simulink model "power_PVArray_PartialShading9x9new"  (R2019a)
settings: Solver=VariableStepAuto  StartTime=0.0  StopTime=9  FixedStep=Ts_Power  RelTol=1e-4
PreLoadFcn:
  | Ts_Power=50e-6;
  | Slope_Vdc=1;
InitFcn:
  | Ts_Power=50e-6;
  | Tc=1e-5;%break algebraic loop time constant
  | BlockName=[gcs,'/PV module 1'];
  | ModuleName=get_param(BlockName,'ModuleName');
  | Voc1=str2num(get_param(BlockName,'Voc'));
  | Nser1=str2num(get_param(BlockName,'Nser'));
  | Slope_Vdc=Nser1*Voc1;
StopFcn:
  | if exist('I','var') && exist('V','var')
  |    figure(1)
  |    clf
  |    n=find(I>=0);
  |    n=n(end);
  |    Vglobal=V(1:n);
  |    Iglobal=I(1:n);
  | 
  | 
  |    Pglobal=Vglobal.*Iglobal;
  |    n=find(Pglobal==max(Pglobal));
  |    Pmax=Pglobal(n);
  |    Vmp=Vglobal(n);
  |    Imp=Iglobal(n);
  | 
  | 
  |    subplot(211)
  |    plot(Vglobal, Iglobal,Vmp,Imp,'or')
  |    ylabel('Current (A)')
  |    title(sprintf('Global I-V & P-V characteristics\n %s' ,ModuleName))
  | 
  | 
  |    subplot(212)
  |    plot(Vglobal, Pglobal,Vmp,Pmax,'or')
  |    ylabel('Power (W)')
  |    xlabel('Voltage (V)')
  | end
undefined symbols (not defined in the file or in its folder): Irr
libraries: powerlib x85, re_lib x81, simulink x1
Description:
  | Copyright 2008-2019 The MathWorks, Inc.
settings Model: Creator=MathWorks  LastModifiedBy=makis
settings SolverCC: AlgebraicLoopSolver=LineSearch
settings DataIOCC: LimitDataPoints=on  SaveFormat=Array  SignalLoggingSaveFormat=ModelDataLogs  ReturnWorkspaceOutputs=off
settings OptimizationCC: ExpressionDepthLimit=2147483647  LifeSpan=inf
settings DebuggingCC: UnderspecifiedInitializationDetection=Classic  MergeDetectMultiDrivingBlocksExec=none  SolverPrmCheckMsg=warning  FcnCallInpInsideContextMsg=warning  AllowSymbolicDim=off  StateNameClashWarn=warning  SFUnexpectedBacktrackingDiag=warning  SFNoUnconditionalDefaultTransitionDiag=warning  SFExecutionAtInitializationDiag=none  ArithmeticOperatorsInVariantConditions=warning
settings HardwareCC: ProdBitPerPointer=32  ProdBitPerSizeT=32  ProdBitPerPtrDiffT=32  ProdLargestAtomicFloat=None  ProdIntDivRoundTo=Undefined  ProdEndianess=Unspecified  ProdWordSize=32  ProdHWDeviceType=32-bit Generic
settings ModelReferenceCC: PropagateSignalLabelsOutOfModel=off
settings SFSimCC: SimUseLocalCustomCode=off
settings RTWCC: RTWUseLocalCustomCode=off
settings CodeAppCC: StateflowObjectComments=on
settings GRTTargetCC: TargetLangStandard=C89/C90 (ANSI)  GeneratePreprocessorConditionals=Disable all  CombineOutputUpdateFcns=off  GRTInterface=on
settings ConfigComp: CovMetricSettings=dw  CovHtmlReporting=on  CovSaveCumulativeToWorkspaceVar=on  CovSaveSingleToWorkspaceVar=on  CovExternalEMLEnable=off  CovSFcnEnable=off
settings SimscapeCC: SimscapeNormalizeSystem=off

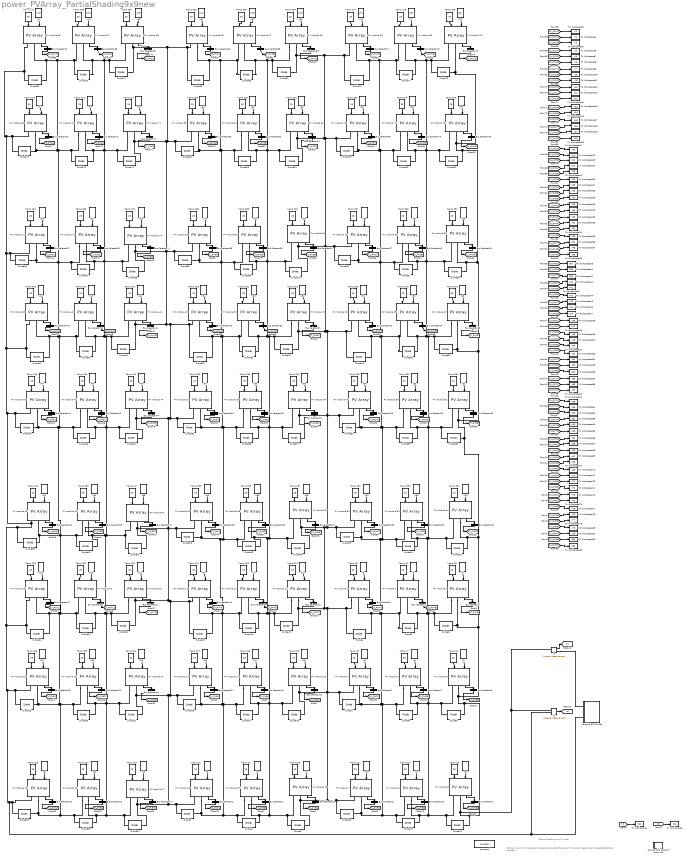
== system power_PVArray_PartialShading9x9new ==
  note: Global I-V and P-V characteristic are displayed at the end of simulation
      | (see Model Properties/Callback StopFcn)
  note: Partial Shading of a PV Array
  Bus Selector{1..81} (81 alike) : BusSelector  OutputSignals=V_PV,I_PV  OutputAsBus=on
  Diode{1..81} (81 alike) : powerlib/Power Electronics/Diode  Ron=0.001  Lon=0  Vf=0.7  IC=0  UseSnubber=off  Rs=1e5*inf  Cs=inf  Measurements=off
      settings: SourceProductName=Simscape Electrical
  Double click here for more info : Subsystem
      settings: OpenFcn=showdemo(bdroot(gcb))
      mask Display: disp('?')
  I1 : powerlib/Measurements/Current Measurement  PhasorSimulation=off  OutputType=Complex  PSBequivalent=0
      settings: SourceProductName=Simscape Electrical
  Ir1 : Constant  Value=Irr(78)
  Ir10 : Constant  Value=Irr(81)
  Ir11 : Constant  Value=Irr(80)
  Ir12 : Constant  Value=Irr(79)
  Ir13 : Constant  Value=Irr(60)
  Ir14 : Constant  Value=Irr(59)
  Ir15 : Constant  Value=Irr(58)
  Ir16 : Constant  Value=Irr(69)
  Ir17 : Constant  Value=Irr(68)
  Ir18 : Constant  Value=Irr(67)
  Ir19 : Constant  Value=Irr(75)
  Ir2 : Constant  Value=Irr(77)
  Ir20 : Constant  Value=Irr(74)
  Ir21 : Constant  Value=Irr(73)
  Ir22 : Constant  Value=Irr(57)
  Ir23 : Constant  Value=Irr(56)
  Ir24 : Constant  Value=Irr(55)
  Ir25 : Constant  Value=Irr(66)
  Ir26 : Constant  Value=Irr(65)
  Ir27 : Constant  Value=Irr(64)
  Ir28 : Constant  Value=Irr(51)
  Ir29 : Constant  Value=Irr(54)
  Ir3 : Constant  Value=Irr(76)
  Ir30 : Constant  Value=Irr(53)
  Ir31 : Constant  Value=Irr(52)
  Ir32 : Constant  Value=Irr(33)
  Ir33 : Constant  Value=Irr(32)
  Ir34 : Constant  Value=Irr(31)
  Ir35 : Constant  Value=Irr(42)
  Ir36 : Constant  Value=Irr(41)
  Ir37 : Constant  Value=Irr(40)
  Ir38 : Constant  Value=Irr(48)
  Ir39 : Constant  Value=Irr(50)
  Ir4 : Constant  Value=Irr(63)
  Ir40 : Constant  Value=Irr(47)
  Ir41 : Constant  Value=Irr(46)
  Ir42 : Constant  Value=Irr(30)
  Ir43 : Constant  Value=Irr(29)
  Ir44 : Constant  Value=Irr(28)
  Ir45 : Constant  Value=Irr(39)
  Ir46 : Constant  Value=Irr(38)
  Ir47 : Constant  Value=Irr(37)
  Ir48 : Constant  Value=Irr(49)
  Ir49 : Constant  Value=Irr(36)
  Ir5 : Constant  Value=Irr(62)
  Ir50 : Constant  Value=Irr(35)
  Ir51 : Constant  Value=Irr(34)
  Ir52 : Constant  Value=Irr(45)
  Ir53 : Constant  Value=Irr(44)
  Ir54 : Constant  Value=Irr(43)
  Ir55 : Constant  Value=Irr(24)
  Ir56 : Constant  Value=Irr(27)
  Ir57 : Constant  Value=Irr(26)
  Ir58 : Constant  Value=Irr(25)
  Ir59 : Constant  Value=Irr(6)
  Ir6 : Constant  Value=Irr(61)
  Ir60 : Constant  Value=Irr(5)
  Ir61 : Constant  Value=Irr(4)
  Ir62 : Constant  Value=Irr(15)
  Ir63 : Constant  Value=Irr(14)
  Ir64 : Constant  Value=Irr(13)
  Ir65 : Constant  Value=Irr(21)
  Ir66 : Constant  Value=Irr(23)
  Ir67 : Constant  Value=Irr(20)
  Ir68 : Constant  Value=Irr(19)
  Ir69 : Constant  Value=Irr(3)
  Ir7 : Constant  Value=Irr(72)
  Ir70 : Constant  Value=Irr(2)
  Ir71 : Constant  Value=Irr(1)
  Ir72 : Constant  Value=Irr(12)
  Ir73 : Constant  Value=Irr(11)
  Ir74 : Constant  Value=Irr(10)
  Ir75 : Constant  Value=Irr(22)
  Ir76 : Constant  Value=Irr(9)
  Ir77 : Constant  Value=Irr(8)
  Ir78 : Constant  Value=Irr(7)
  Ir79 : Constant  Value=Irr(18)
  Ir8 : Constant  Value=Irr(71)
  Ir80 : Constant  Value=Irr(17)
  Ir81 : Constant  Value=Irr(16)
  Ir9 : Constant  Value=Irr(70)
  PV module {1..81} (81 alike) : re_lib/Solar/PV Array  Npar=1  Nser=1  PlotType=array @ 25 deg.C & specified irradiances  S_vec="[ 1000  500  100 ]"  Temp_C_vec="[ 45 25  ]"  ModuleName=Mitsubishi Electric PV-MLU255HC  PlotWhenSelected=off  Pm=255.216  Ncell=60  Voc=37.8  Isc=8.89  Vm=31.2  Im=8.18  beta_Voc_pc=-0.38701  alpha_Isc_pc=0.104  beta_Voc=-0.14629  alpha_Isc=0.009246  IL=8.9065  I0=7.8419e-10  nI=1.0608  Rsh=114.9388  Rs=0.21303  BAL=on  Tc=Tc  Tfilter=5e-5
      settings: SourceProductName=Simscape Electrical
  Temp C{1..81} (81 alike) : Constant  Value=25
  To Workspace1 : ToWorkspace  VariableName=Vtot  SampleTime=1e-3
  To Workspace10 : ToWorkspace  VariableName=V8  SampleTime=1e-3
  To Workspace11 : ToWorkspace  VariableName=V9  SampleTime=1e-3
  To Workspace12 : ToWorkspace  VariableName=V10  SampleTime=1e-3
  To Workspace13 : ToWorkspace  VariableName=V11  SampleTime=1e-3
  To Workspace14 : ToWorkspace  VariableName=V12  SampleTime=1e-3
  To Workspace15 : ToWorkspace  VariableName=V13  SampleTime=1e-3
  To Workspace16 : ToWorkspace  VariableName=V14  SampleTime=1e-3
  To Workspace17 : ToWorkspace  VariableName=V15  SampleTime=1e-3
  To Workspace18 : ToWorkspace  VariableName=V16  SampleTime=1e-3
  To Workspace19 : ToWorkspace  VariableName=V17  SampleTime=1e-3
  To Workspace2 : ToWorkspace  VariableName=Itot  SampleTime=1e-3
  To Workspace20 : ToWorkspace  VariableName=V18  SampleTime=1e-3
  To Workspace21 : ToWorkspace  VariableName=V19  SampleTime=1e-3
  To Workspace22 : ToWorkspace  VariableName=V20  SampleTime=1e-3
  To Workspace23 : ToWorkspace  VariableName=V21  SampleTime=1e-3
  To Workspace24 : ToWorkspace  VariableName=V22  SampleTime=1e-3
  To Workspace25 : ToWorkspace  VariableName=V23  SampleTime=1e-3
  To Workspace26 : ToWorkspace  VariableName=V24  SampleTime=1e-3
  To Workspace27 : ToWorkspace  VariableName=V25  SampleTime=1e-3
  To Workspace28 : ToWorkspace  VariableName=V26  SampleTime=1e-3
  To Workspace29 : ToWorkspace  VariableName=V27  SampleTime=1e-3
  To Workspace3 : ToWorkspace  VariableName=V1  SampleTime=1e-3
  To Workspace30 : ToWorkspace  VariableName=V28  SampleTime=1e-3
  To Workspace31 : ToWorkspace  VariableName=V29  SampleTime=1e-3
  To Workspace32 : ToWorkspace  VariableName=V30  SampleTime=1e-3
  To Workspace33 : ToWorkspace  VariableName=V31  SampleTime=1e-3
  To Workspace34 : ToWorkspace  VariableName=V32  SampleTime=1e-3
  To Workspace35 : ToWorkspace  VariableName=V33  SampleTime=1e-3
  To Workspace36 : ToWorkspace  VariableName=V34  SampleTime=1e-3
  To Workspace37 : ToWorkspace  VariableName=V35  SampleTime=1e-3
  To Workspace38 : ToWorkspace  VariableName=V36  SampleTime=1e-3
  To Workspace39 : ToWorkspace  VariableName=V37  SampleTime=1e-3
  To Workspace4 : ToWorkspace  VariableName=V2  SampleTime=1e-3
  To Workspace40 : ToWorkspace  VariableName=V38  SampleTime=1e-3
  To Workspace41 : ToWorkspace  VariableName=V39  SampleTime=1e-3
  To Workspace42 : ToWorkspace  VariableName=V40  SampleTime=1e-3
  To Workspace43 : ToWorkspace  VariableName=V41  SampleTime=1e-3
  To Workspace44 : ToWorkspace  VariableName=V42  SampleTime=1e-3
  To Workspace45 : ToWorkspace  VariableName=V43  SampleTime=1e-3
  To Workspace46 : ToWorkspace  VariableName=V44  SampleTime=1e-3
  To Workspace47 : ToWorkspace  VariableName=V45  SampleTime=1e-3
  To Workspace48 : ToWorkspace  VariableName=V46  SampleTime=1e-3
  To Workspace49 : ToWorkspace  VariableName=V47  SampleTime=1e-3
  To Workspace5 : ToWorkspace  VariableName=V3  SampleTime=1e-3
  To Workspace50 : ToWorkspace  VariableName=V48  SampleTime=1e-3
  To Workspace51 : ToWorkspace  VariableName=V49  SampleTime=1e-3
  To Workspace52 : ToWorkspace  VariableName=V50  SampleTime=1e-3
  To Workspace53 : ToWorkspace  VariableName=V51  SampleTime=1e-3
  To Workspace54 : ToWorkspace  VariableName=V52  SampleTime=1e-3
  To Workspace55 : ToWorkspace  VariableName=V53  SampleTime=1e-3
  To Workspace56 : ToWorkspace  VariableName=V54  SampleTime=1e-3
  To Workspace57 : ToWorkspace  VariableName=V55  SampleTime=1e-3
  To Workspace58 : ToWorkspace  VariableName=V56  SampleTime=1e-3
  To Workspace59 : ToWorkspace  VariableName=V57  SampleTime=1e-3
  To Workspace6 : ToWorkspace  VariableName=V4  SampleTime=1e-3
  To Workspace60 : ToWorkspace  VariableName=V58  SampleTime=1e-3
  To Workspace61 : ToWorkspace  VariableName=V59  SampleTime=1e-3
  To Workspace62 : ToWorkspace  VariableName=V60  SampleTime=1e-3
  To Workspace63 : ToWorkspace  VariableName=V61  SampleTime=1e-3
  To Workspace64 : ToWorkspace  VariableName=V62  SampleTime=1e-3
  To Workspace65 : ToWorkspace  VariableName=V63  SampleTime=1e-3
  To Workspace66 : ToWorkspace  VariableName=V64  SampleTime=1e-3
  To Workspace67 : ToWorkspace  VariableName=V65  SampleTime=1e-3
  To Workspace68 : ToWorkspace  VariableName=V66  SampleTime=1e-3
  To Workspace69 : ToWorkspace  VariableName=V67  SampleTime=1e-3
  To Workspace7 : ToWorkspace  VariableName=V5  SampleTime=1e-3
  To Workspace70 : ToWorkspace  VariableName=V68  SampleTime=1e-3
  To Workspace71 : ToWorkspace  VariableName=V69  SampleTime=1e-3
  To Workspace72 : ToWorkspace  VariableName=V70  SampleTime=1e-3
  To Workspace73 : ToWorkspace  VariableName=V71  SampleTime=1e-3
  To Workspace74 : ToWorkspace  VariableName=V72  SampleTime=1e-3
  To Workspace75 : ToWorkspace  VariableName=V73  SampleTime=1e-3
  To Workspace76 : ToWorkspace  VariableName=V74  SampleTime=1e-3
  To Workspace77 : ToWorkspace  VariableName=V75  SampleTime=1e-3
  To Workspace78 : ToWorkspace  VariableName=V76  SampleTime=1e-3
  To Workspace79 : ToWorkspace  VariableName=V77  SampleTime=1e-3
  To Workspace8 : ToWorkspace  VariableName=V6  SampleTime=1e-3
  To Workspace80 : ToWorkspace  VariableName=V78  SampleTime=1e-3
  To Workspace81 : ToWorkspace  VariableName=V79  SampleTime=1e-3
  To Workspace82 : ToWorkspace  VariableName=V80  SampleTime=1e-3
  To Workspace83 : ToWorkspace  VariableName=V81  SampleTime=1e-3
  To Workspace9 : ToWorkspace  VariableName=V7  SampleTime=1e-3
  V1 : powerlib/Measurements/Voltage Measurement  PhasorSimulation=off  OutputType=Complex  PSBequivalent=0
      settings: SourceProductName=Simscape Electrical
  Variable DC Source1 : Subsystem
  powergui : powerlib/powergui  Priority=1  SimulationMode=Continuous  SampleTime=Ts_Power*0 + 20e-6  frequency=60  Iterations=50  frequencyindice=0  Pbase=100e6  ErrMax=1e-4  UnitsV=kV  UnitsW=MW  buscounter=0  FunctionMessages=off  echomessages=off  EnableUseOfTLC=off  CurrentSourceSwitches=on  DisableSnubberDevices=on  DisableRonSwitches=off  DisableVfSwitches=off  DisplayEquations=off  AutomaticDiscreteSolvers=off  SolverType=Tustin/Backward Euler (TBE)  Interpol=off  ExternalGateDelay=off  methode=off  Ts=0  x0status=blocks  SPID=off  SwTol=0  HookPort=off  NonlinearTolerance=0  nMaxIteration=15  ContinueOnMaxIteration=off  RestoreLinks=warning  ResistiveCurrentMeasurement=off  Frange=[0:2:500]  Ylog=off  Xlog=on  ShowGrid=off  save=off  variable=ZData  structure=0  ZoomFFT=on  StartTime=0.0  cycles=1  DisplayStyle=1  fundamental=60  FreqAxis=off  MaxFrequency=1000  frequencyindicesteady=1  RmsSteady=1  display=off
      settings: SourceProductName=Simscape Electrical
  wires:
  [V] -> To Workspace1/1
  [I] -> To Workspace2/1
  PV module 1/1 -> Bus Selector5/1
  Temp C5/1 -> PV module 1/2
  PV module 3/1 -> Bus Selector3/1
  Ir4/1 -> PV module 3/1
  Bus Selector5/1 -> [VI_PV77]
  PV module 2/1 -> Bus Selector4/1
  Bus Selector3/1 -> [VI_PV79]
  Bus Selector4/1 -> [VI_PV78]
  Ir6/1 -> PV module 1/1
  Ir5/1 -> PV module 2/1
  Temp C4/1 -> PV module 2/2
  Temp C3/1 -> PV module 3/2
  Bus Selector6/1 -> [VI_PV89]
  Temp C6/1 -> PV module 6/2
  Bus Selector7/1 -> [VI_PV88]
  Ir8/1 -> PV module 5/1
  Temp C7/1 -> PV module 5/2
  Ir9/1 -> PV module 4/1
  PV module 4/1 -> Bus Selector8/1
  PV module 5/1 -> Bus Selector7/1
  Ir7/1 -> PV module 6/1
  Bus Selector8/1 -> [VI_PV87]
  PV module 6/1 -> Bus Selector6/1
  Temp C8/1 -> PV module 4/2
  Bus Selector9/1 -> [VI_PV99]
  PV module 8/1 -> Bus Selector10/1
  Ir10/1 -> PV module 9/1
  PV module 7/1 -> Bus Selector11/1
  Temp C10/1 -> PV module 8/2
  Temp C9/1 -> PV module 9/2
  Ir11/1 -> PV module 8/1
  Bus Selector10/1 -> [VI_PV98]
  Ir12/1 -> PV module 7/1
  Temp C11/1 -> PV module 7/2
  Bus Selector11/1 -> [VI_PV97]
  PV module 9/1 -> Bus Selector9/1
  V1/1 -> [V]
  I1/1 -> [I]
  Bus Selector13/1 -> [VI_PV75]
  PV module 16/1 -> Bus Selector2/1
  PV module 17/1 -> Bus Selector1/1
  Ir16/1 -> PV module 15/1
  Temp C16/1 -> PV module 14/2
  Ir2/1 -> PV module 17/1
  PV module 18/1 -> Bus Selector18/1
  Bus Selector2/1 -> [VI_PV94]
  Bus Selector17/1 -> [VI_PV84]
  Temp C2/1 -> PV module 16/2
  Ir3/1 -> PV module 16/1
  Bus Selector1/1 -> [VI_PV95]
  PV module 11/1 -> Bus Selector13/1
  Temp C1/1 -> PV module 17/2
  Temp C18/1 -> PV module 18/2
  Ir1/1 -> PV module 18/1
  Temp C17/1 -> PV module 13/2
  Ir18/1 -> PV module 13/1
  Bus Selector18/1 -> [VI_PV96]
  PV module 14/1 -> Bus Selector16/1
  Ir15/1 -> PV module 10/1
  PV module 13/1 -> Bus Selector17/1
  Ir17/1 -> PV module 14/1
  Ir14/1 -> PV module 11/1
  Temp C15/1 -> PV module 15/2
  Bus Selector15/1 -> [VI_PV86]
  Bus Selector12/1 -> [VI_PV76]
  Bus Selector14/1 -> [VI_PV74]
  Ir13/1 -> PV module 12/1
  PV module 12/1 -> Bus Selector12/1
  Bus Selector16/1 -> [VI_PV85]
  Temp C14/1 -> PV module 10/2
  PV module 10/1 -> Bus Selector14/1
  Temp C13/1 -> PV module 11/2
  PV module 15/1 -> Bus Selector15/1
  Temp C12/1 -> PV module 12/2
  Bus Selector22/1 -> [VI_PV72]
  PV module 25/1 -> Bus Selector20/1
  PV module 26/1 -> Bus Selector19/1
  Ir25/1 -> PV module 24/1
  Temp C25/1 -> PV module 23/2
  Ir20/1 -> PV module 26/1
  PV module 27/1 -> Bus Selector27/1
  Bus Selector20/1 -> [VI_PV91]
  Bus Selector26/1 -> [VI_PV81]
  Temp C20/1 -> PV module 25/2
  Ir21/1 -> PV module 25/1
  Bus Selector19/1 -> [VI_PV92]
  PV module 20/1 -> Bus Selector22/1
  Temp C19/1 -> PV module 26/2
  Temp C27/1 -> PV module 27/2
  Ir19/1 -> PV module 27/1
  Temp C26/1 -> PV module 22/2
  Ir27/1 -> PV module 22/1
  Bus Selector27/1 -> [VI_PV93]
  PV module 23/1 -> Bus Selector25/1
  Ir24/1 -> PV module 19/1
  PV module 22/1 -> Bus Selector26/1
  Ir26/1 -> PV module 23/1
  Ir23/1 -> PV module 20/1
  Temp C24/1 -> PV module 24/2
  Bus Selector24/1 -> [VI_PV83]
  Bus Selector21/1 -> [VI_PV73]
  Bus Selector23/1 -> [VI_PV71]
  Ir22/1 -> PV module 21/1
  PV module 21/1 -> Bus Selector21/1
  Bus Selector25/1 -> [VI_PV82]
  Temp C23/1 -> PV module 19/2
  PV module 19/1 -> Bus Selector23/1
  Temp C22/1 -> PV module 20/2
  PV module 24/1 -> Bus Selector24/1
  Temp C21/1 -> PV module 21/2
  Bus Selector49/1 -> [VI_PV48]
  PV module 52/1 -> Bus Selector30/1
  PV module 53/1 -> Bus Selector29/1
  Bus Selector30/1 -> [VI_PV67]
  Bus Selector53/1 -> [VI_PV57]
  Bus Selector29/1 -> [VI_PV68]
  Ir51/1 -> PV module 28/1
  Temp C48/1 -> PV module 48/2
  Ir31/1 -> PV module 52/1
  Temp C29/1 -> PV module 53/2
  PV module 48/1 -> Bus Selector48/1
  Ir29/1 -> PV module 54/1
  Bus Selector51/1 -> [VI_PV59]
  Temp C53/1 -> PV module 49/2
  PV module 51/1 -> Bus Selector51/1
  PV module 50/1 -> Bus Selector52/1
  PV module 49/1 -> Bus Selector53/1
  Ir53/1 -> PV module 50/1
  Bus Selector52/1 -> [VI_PV58]
  Temp C51/1 -> PV module 51/2
  Temp C49/1 -> PV module 39/2
  Ir50/1 -> PV module 39/1
  Bus Selector48/1 -> [VI_PV49]
  Bus Selector50/1 -> [VI_PV47]
  Ir49/1 -> PV module 48/1
  Temp C50/1 -> PV module 28/2
  PV module 28/1 -> Bus Selector50/1
  Temp C41/1 -> PV module 41/2
  PV module 44/1 -> Bus Selector44/1
  Temp C42/1 -> PV module 40/2
  Temp C43/1 -> PV module 38/2
  PV module 41/1 -> Bus Selector41/1
  Ir42/1 -> PV module 41/1
  Bus Selector41/1 -> [VI_PV43]
  Temp C44/1 -> PV module 44/2
  Ir46/1 -> PV module 43/1
  PV module 42/1 -> Bus Selector46/1
  Ir44/1 -> PV module 38/1
  PV module 43/1 -> Bus Selector45/1
  Bus Selector47/1 -> [VI_PV63]
  Ir47/1 -> PV module 42/1
  Temp C46/1 -> PV module 42/2
  Ir38/1 -> PV module 47/1
  Temp C38/1 -> PV module 46/2
  PV module 40/1 -> Bus Selector42/1
  Bus Selector38/1 -> [VI_PV62]
  Ir41/1 -> PV module 45/1
  Temp C40/1 -> PV module 45/2
  PV module 47/1 -> Bus Selector47/1
  Ir40/1 -> PV module 46/1
  Temp C45/1 -> PV module 43/2
  Ir45/1 -> PV module 44/1
  PV module 46/1 -> Bus Selector38/1
  Bus Selector42/1 -> [VI_PV42]
  Temp C54/1 -> PV module 54/2
  PV module 39/1 -> Bus Selector49/1
  Temp C30/1 -> PV module 52/2
  PV module 45/1 -> Bus Selector40/1
  Ir30/1 -> PV module 53/1
  Bus Selector43/1 -> [VI_PV41]
  Ir43/1 -> PV module 40/1
  Ir54/1 -> PV module 49/1
  Temp C31/1 -> PV module 31/2
  PV module 34/1 -> Bus Selector34/1
  Temp C32/1 -> PV module 30/2
  PV module 29/1 -> Bus Selector33/1
  Temp C33/1 -> PV module 29/2
  Bus Selector35/1 -> [VI_PV55]
  PV module 31/1 -> Bus Selector31/1
  Temp C47/1 -> PV module 47/2
  Ir32/1 -> PV module 31/1
  Bus Selector33/1 -> [VI_PV44]
  Bus Selector31/1 -> [VI_PV46]
  Bus Selector34/1 -> [VI_PV56]
  Temp C34/1 -> PV module 34/2
  Ir33/1 -> PV module 30/1
  PV module 33/1 -> Bus Selector35/1
  Bus Selector37/1 -> [VI_PV66]
  Temp C36/1 -> PV module 32/2
  Ir37/1 -> PV module 32/1
  Ir28/1 -> PV module 37/1
  Temp C37/1 -> PV module 37/2
  Ir36/1 -> PV module 33/1
  Bus Selector46/1 -> [VI_PV51]
  Ir34/1 -> PV module 29/1
  PV module 32/1 -> Bus Selector36/1
  Bus Selector40/1 -> [VI_PV61]
  PV module 38/1 -> Bus Selector43/1
  Temp C52/1 -> PV module 50/2
  Bus Selector32/1 -> [VI_PV45]
  PV module 35/1 -> Bus Selector39/1
  Bus Selector44/1 -> [VI_PV53]
  PV module 36/1 -> Bus Selector28/1
  Bus Selector54/1 -> [VI_PV69]
  Ir35/1 -> PV module 34/1
  Temp C35/1 -> PV module 33/2
  Ir39/1 -> PV module 36/1
  PV module 37/1 -> Bus Selector37/1
  Bus Selector39/1 -> [VI_PV64]
  Bus Selector36/1 -> [VI_PV54]
  Temp C39/1 -> PV module 35/2
  Ir52/1 -> PV module 51/1
  Ir48/1 -> PV module 35/1
  Bus Selector28/1 -> [VI_PV65]
  PV module 30/1 -> Bus Selector32/1
  Temp C28/1 -> PV module 36/2
  Bus Selector45/1 -> [VI_PV52]
  PV module 54/1 -> Bus Selector54/1
  Bus Selector76/1 -> [VI_PV18]
  PV module 79/1 -> Bus Selector57/1
  PV module 80/1 -> Bus Selector56/1
  Bus Selector57/1 -> [VI_PV37]
  Bus Selector80/1 -> [VI_PV27]
  Bus Selector56/1 -> [VI_PV38]
  Ir78/1 -> PV module 55/1
  Temp C75/1 -> PV module 75/2
  Ir58/1 -> PV module 79/1
  Temp C56/1 -> PV module 80/2
  PV module 75/1 -> Bus Selector75/1
  Ir56/1 -> PV module 81/1
  Bus Selector78/1 -> [VI_PV29]
  Temp C80/1 -> PV module 76/2
  PV module 78/1 -> Bus Selector78/1
  PV module 77/1 -> Bus Selector79/1
  PV module 76/1 -> Bus Selector80/1
  Ir80/1 -> PV module 77/1
  Bus Selector79/1 -> [VI_PV28]
  Temp C78/1 -> PV module 78/2
  Temp C76/1 -> PV module 66/2
  Ir77/1 -> PV module 66/1
  Bus Selector75/1 -> [VI_PV19]
  Bus Selector77/1 -> [VI_PV17]
  Ir76/1 -> PV module 75/1
  Temp C77/1 -> PV module 55/2
  PV module 55/1 -> Bus Selector77/1
  Temp C68/1 -> PV module 68/2
  PV module 71/1 -> Bus Selector71/1
  Temp C69/1 -> PV module 67/2
  Temp C70/1 -> PV module 65/2
  PV module 68/1 -> Bus Selector68/1
  Ir69/1 -> PV module 68/1
  Bus Selector68/1 -> [VI_PV13]
  Temp C71/1 -> PV module 71/2
  Ir73/1 -> PV module 70/1
  PV module 69/1 -> Bus Selector73/1
  Ir71/1 -> PV module 65/1
  PV module 70/1 -> Bus Selector72/1
  Bus Selector74/1 -> [VI_PV33]
  Ir74/1 -> PV module 69/1
  Temp C73/1 -> PV module 69/2
  Ir65/1 -> PV module 74/1
  Temp C65/1 -> PV module 73/2
  PV module 67/1 -> Bus Selector69/1
  Bus Selector65/1 -> [VI_PV32]
  Ir68/1 -> PV module 72/1
  Temp C67/1 -> PV module 72/2
  PV module 74/1 -> Bus Selector74/1
  Ir67/1 -> PV module 73/1
  Temp C72/1 -> PV module 70/2
  Ir72/1 -> PV module 71/1
  PV module 73/1 -> Bus Selector65/1
  Bus Selector69/1 -> [VI_PV12]
  Temp C81/1 -> PV module 81/2
  PV module 66/1 -> Bus Selector76/1
  Temp C57/1 -> PV module 79/2
  PV module 72/1 -> Bus Selector67/1
  Ir57/1 -> PV module 80/1
  Bus Selector70/1 -> [VI_PV11]
  Ir70/1 -> PV module 67/1
  Ir81/1 -> PV module 76/1
  Temp C58/1 -> PV module 58/2
  PV module 61/1 -> Bus Selector61/1
  Temp C59/1 -> PV module 57/2
  PV module 56/1 -> Bus Selector60/1
  Temp C60/1 -> PV module 56/2
  Bus Selector62/1 -> [VI_PV25]
  PV module 58/1 -> Bus Selector58/1
  Temp C74/1 -> PV module 74/2
  Ir59/1 -> PV module 58/1
  Bus Selector60/1 -> [VI_PV14]
  Bus Selector58/1 -> [VI_PV16]
  Bus Selector61/1 -> [VI_PV26]
  Temp C61/1 -> PV module 61/2
  Ir60/1 -> PV module 57/1
  PV module 60/1 -> Bus Selector62/1
  Bus Selector64/1 -> [VI_PV36]
  Temp C63/1 -> PV module 59/2
  Ir64/1 -> PV module 59/1
  Ir55/1 -> PV module 64/1
  Temp C64/1 -> PV module 64/2
  Ir63/1 -> PV module 60/1
  Bus Selector73/1 -> [VI_PV21]
  Ir61/1 -> PV module 56/1
  PV module 59/1 -> Bus Selector63/1
  Bus Selector67/1 -> [VI_PV31]
  PV module 65/1 -> Bus Selector70/1
  Temp C79/1 -> PV module 77/2
  Bus Selector59/1 -> [VI_PV15]
  PV module 62/1 -> Bus Selector66/1
  Bus Selector71/1 -> [VI_PV23]
  PV module 63/1 -> Bus Selector55/1
  Bus Selector81/1 -> [VI_PV39]
  Ir62/1 -> PV module 61/1
  Temp C62/1 -> PV module 60/2
  Ir66/1 -> PV module 63/1
  PV module 64/1 -> Bus Selector64/1
  Bus Selector66/1 -> [VI_PV34]
  Bus Selector63/1 -> [VI_PV24]
  Temp C66/1 -> PV module 62/2
  Ir79/1 -> PV module 78/1
  Ir75/1 -> PV module 62/1
  Bus Selector55/1 -> [VI_PV35]
  PV module 57/1 -> Bus Selector59/1
  Temp C55/1 -> PV module 63/2
  Bus Selector72/1 -> [VI_PV22]
  PV module 81/1 -> Bus Selector81/1
  [VI_PV26] -> To Workspace17/1
  [VI_PV86] -> To Workspace71/1
  [VI_PV96] -> To Workspace80/1
  [VI_PV48] -> To Workspace37/1
  [VI_PV81] -> To Workspace66/1
  [VI_PV35] -> To Workspace25/1
  [VI_PV39] -> To Workspace29/1
  [VI_PV75] -> To Workspace61/1
  [VI_PV45] -> To Workspace34/1
  [VI_PV68] -> To Workspace55/1
  [VI_PV87] -> To Workspace72/1
  [VI_PV72] -> To Workspace58/1
  [VI_PV71] -> To Workspace57/1
  [VI_PV63] -> To Workspace50/1
  [VI_PV28] -> To Workspace19/1
  [VI_PV74] -> To Workspace60/1
  [VI_PV91] -> To Workspace75/1
  [VI_PV46] -> To Workspace35/1
  [VI_PV65] -> To Workspace52/1
  [VI_PV79] -> To Workspace65/1
  [VI_PV77] -> To Workspace63/1
  [VI_PV49] -> To Workspace38/1
  [VI_PV93] -> To Workspace77/1
  [VI_PV69] -> To Workspace56/1
  [VI_PV85] -> To Workspace70/1
  [VI_PV44] -> To Workspace33/1
  [VI_PV59] -> To Workspace47/1
  [VI_PV47] -> To Workspace36/1
  [VI_PV54] -> To Workspace42/1
  [VI_PV21] -> To Workspace12/1
  [VI_PV43] -> To Workspace32/1
  [VI_PV22] -> To Workspace13/1
  [VI_PV34] -> To Workspace24/1
  [VI_PV38] -> To Workspace28/1
  [VI_PV37] -> To Workspace27/1
  [VI_PV23] -> To Workspace14/1
  [VI_PV51] -> To Workspace39/1
  [VI_PV53] -> To Workspace41/1
  [VI_PV56] -> To Workspace44/1
  [VI_PV27] -> To Workspace18/1
  [VI_PV33] -> To Workspace23/1
  [VI_PV67] -> To Workspace54/1
  [VI_PV31] -> To Workspace21/1
  [VI_PV42] -> To Workspace31/1
  [VI_PV41] -> To Workspace30/1
  [VI_PV36] -> To Workspace26/1
  [VI_PV76] -> To Workspace62/1
  [VI_PV89] -> To Workspace74/1
  [VI_PV52] -> To Workspace40/1
  [VI_PV24] -> To Workspace15/1
  [VI_PV55] -> To Workspace43/1
  [VI_PV57] -> To Workspace45/1
  [VI_PV58] -> To Workspace46/1
  [VI_PV62] -> To Workspace49/1
  [VI_PV61] -> To Workspace48/1
  [VI_PV66] -> To Workspace53/1
  [VI_PV73] -> To Workspace59/1
  [VI_PV82] -> To Workspace67/1
  [VI_PV88] -> To Workspace73/1
  [VI_PV95] -> To Workspace79/1
  [VI_PV29] -> To Workspace20/1
  [VI_PV84] -> To Workspace69/1
  [VI_PV83] -> To Workspace68/1
  [VI_PV64] -> To Workspace51/1
  [VI_PV97] -> To Workspace81/1
  [VI_PV32] -> To Workspace22/1
  [VI_PV98] -> To Workspace82/1
  [VI_PV92] -> To Workspace76/1
  [VI_PV78] -> To Workspace64/1
  [VI_PV94] -> To Workspace78/1
  [VI_PV99] -> To Workspace83/1
  [VI_PV25] -> To Workspace16/1
  [VI_PV19] -> To Workspace11/1
  [VI_PV18] -> To Workspace10/1
  [VI_PV17] -> To Workspace9/1
  [VI_PV16] -> To Workspace8/1
  [VI_PV15] -> To Workspace7/1
  [VI_PV14] -> To Workspace6/1
  [VI_PV13] -> To Workspace5/1
  [VI_PV12] -> To Workspace4/1
  [VI_PV11] -> To Workspace3/1
  connections:
  PV module 55/RConn1 -- Diode76/RConn1 -- PV module 66/RConn2 -- Diode77/LConn1 -- Diode79/RConn1 -- PV module 76/RConn1 -- Diode80/LConn1 -- PV module 77/RConn2 -- Diode56/RConn1 -- PV module 79/RConn1 -- PV module 39/RConn2 -- Diode50/LConn1 -- Diode52/RConn1 -- PV module 49/RConn1 -- Diode53/LConn1 -- PV module 50/RConn2 -- Diode29/RConn1 -- PV module 52/RConn1 -- PV module 1/RConn1 -- Diode4/RConn1 -- PV module 2/RConn2 -- Diode5/LConn1 -- PV module 7/RConn1 -- Diode10/RConn1 -- PV module 8/RConn2 -- Diode11/LConn1 -- Diode8/LConn1 -- PV module 5/RConn2 -- Diode7/RConn1 -- PV module 4/RConn1 -- PV module 53/RConn2 -- Diode30/LConn1 -- PV module 28/RConn1 -- Diode49/RConn1 -- PV module 80/RConn2 -- Diode57/LConn1
  Diode78/LConn1 -- Diode57/RConn1 -- PV module 80/RConn1 -- PV module 39/RConn1 -- Diode50/RConn1 -- PV module 48/RConn2 -- Diode51/LConn1 -- Diode30/RConn1 -- PV module 53/RConn1 -- PV module 2/RConn1 -- Diode5/RConn1 -- PV module 3/RConn2 -- Diode6/LConn1 -- PV module 9/RConn2 -- Diode12/LConn1 -- Diode11/RConn1 -- PV module 8/RConn1 -- Diode8/RConn1 -- PV module 5/RConn1 -- Diode9/LConn1 -- PV module 6/RConn2 -- PV module 54/RConn2 -- Diode31/LConn1 -- Diode53/RConn1 -- PV module 50/RConn1 -- Diode54/LConn1 -- PV module 51/RConn2 -- PV module 81/RConn2 -- Diode58/LConn1 -- Diode80/RConn1 -- PV module 77/RConn1 -- Diode81/LConn1 -- PV module 78/RConn2 -- PV module 66/RConn1 -- Diode77/RConn1 -- PV module 75/RConn2
  I1/RConn1 -- Variable DC Source1/LConn1
  Diode81/RConn1 -- Diode58/RConn1 -- PV module 81/RConn1 -- PV module 51/RConn1 -- Diode54/RConn1 -- Diode31/RConn1 -- PV module 54/RConn1 -- PV module 6/RConn1 -- Diode9/RConn1 -- I1/LConn1 -- V1/LConn1 -- PV module 9/RConn1 -- Diode12/RConn1 -- PV module 3/RConn1 -- Diode6/RConn1 -- PV module 48/RConn1 -- Diode51/RConn1 -- PV module 78/RConn1 -- PV module 75/RConn1 -- Diode78/RConn1
  Diode66/LConn1 -- PV module 63/RConn2 -- Diode55/RConn1 -- PV module 62/RConn1 -- Diode63/LConn1 -- PV module 60/RConn2 -- Diode62/RConn1 -- PV module 59/RConn1 -- PV module 57/RConn2 -- Diode60/LConn1 -- PV module 56/RConn1 -- Diode59/RConn1 -- PV module 29/RConn1 -- Diode32/RConn1 -- PV module 30/RConn2 -- Diode33/LConn1 -- Diode35/RConn1 -- PV module 32/RConn1 -- Diode36/LConn1 -- PV module 33/RConn2 -- Diode28/RConn1 -- PV module 35/RConn1 -- PV module 11/RConn2 -- Diode14/LConn1 -- PV module 10/RConn1 -- Diode13/RConn1 -- Diode16/RConn1 -- PV module 13/RConn1 -- Diode17/LConn1 -- PV module 14/RConn2 -- PV module 16/RConn1 -- Diode1/RConn1 -- PV module 17/RConn2 -- Diode2/LConn1 -- PV module 36/RConn2 -- Diode39/LConn1
  Diode60/RConn1 -- PV module 57/RConn1 -- PV module 58/RConn2 -- Diode61/LConn1 -- Diode63/RConn1 -- PV module 60/RConn1 -- Diode64/LConn1 -- PV module 61/RConn2 -- Diode66/RConn1 -- PV module 63/RConn1 -- PV module 30/RConn1 -- Diode33/RConn1 -- PV module 31/RConn2 -- Diode34/LConn1 -- Diode36/RConn1 -- PV module 33/RConn1 -- Diode37/LConn1 -- PV module 34/RConn2 -- Diode39/RConn1 -- PV module 36/RConn1 -- PV module 12/RConn2 -- Diode15/LConn1 -- Diode17/RConn1 -- PV module 14/RConn1 -- Diode18/LConn1 -- PV module 15/RConn2 -- Diode2/RConn1 -- PV module 17/RConn1 -- PV module 18/RConn2 -- Diode3/LConn1 -- PV module 11/RConn1 -- Diode14/RConn1 -- PV module 37/RConn2 -- Diode48/LConn1 -- PV module 64/RConn2 -- Diode75/LConn1
  Diode72/LConn1 -- PV module 69/RConn2 -- Diode69/LConn1 -- PV module 65/RConn2 -- Diode65/LConn1 -- PV module 72/RConn2 -- Diode42/LConn1 -- PV module 38/RConn2 -- Diode38/LConn1 -- Diode22/LConn1 -- PV module 19/RConn2 -- Variable DC Source1/LConn2 -- V1/LConn2 -- PV module 25/RConn2 -- Diode19/LConn1 -- PV module 22/RConn2 -- Diode25/LConn1 -- PV module 45/RConn2 -- PV module 42/RConn2 -- Diode45/LConn1
  Diode70/RConn1 -- PV module 67/RConn1 -- PV module 68/RConn2 -- Diode71/LConn1 -- Diode73/RConn1 -- PV module 70/RConn1 -- Diode74/LConn1 -- PV module 71/RConn2 -- Diode67/RConn1 -- PV module 73/RConn1 -- PV module 41/RConn2 -- Diode44/LConn1 -- Diode40/RConn1 -- PV module 46/RConn1 -- PV module 20/RConn1 -- Diode23/RConn1 -- PV module 21/RConn2 -- Diode24/LConn1 -- Diode26/RConn1 -- PV module 23/RConn1 -- Diode27/LConn1 -- PV module 24/RConn2 -- Diode20/RConn1 -- PV module 26/RConn1 -- PV module 27/RConn2 -- Diode21/LConn1 -- PV module 47/RConn2 -- Diode41/LConn1 -- Diode46/RConn1 -- PV module 43/RConn1 -- Diode47/LConn1 -- PV module 44/RConn2 -- Diode43/RConn1 -- PV module 40/RConn1 -- PV module 74/RConn2 -- Diode68/LConn1
  Diode62/LConn1 -- PV module 59/RConn2 -- PV module 68/RConn1 -- Diode71/RConn1 -- PV module 56/RConn2 -- Diode59/LConn1 -- PV module 74/RConn1 -- Diode68/RConn1 -- Diode32/LConn1 -- PV module 29/RConn2 -- PV module 32/RConn2 -- Diode35/LConn1 -- Diode24/RConn1 -- PV module 21/RConn1 -- Diode13/LConn1 -- PV module 10/RConn2 -- PV module 27/RConn1 -- Diode21/RConn1 -- Diode1/LConn1 -- PV module 16/RConn2 -- PV module 24/RConn1 -- Diode27/RConn1 -- PV module 13/RConn2 -- Diode16/LConn1 -- PV module 47/RConn1 -- Diode41/RConn1 -- Diode28/LConn1 -- PV module 35/RConn2 -- PV module 44/RConn1 -- Diode47/RConn1 -- Diode44/RConn1 -- PV module 41/RConn1 -- PV module 62/RConn2 -- Diode55/LConn1 -- PV module 71/RConn1 -- Diode74/RConn1
  PV module 79/RConn2 -- Diode56/LConn1 -- PV module 64/RConn1 -- Diode75/RConn1 -- Diode49/LConn1 -- PV module 28/RConn2 -- Diode37/RConn1 -- PV module 34/RConn1 -- Diode52/LConn1 -- PV module 49/RConn2 -- Diode48/RConn1 -- PV module 37/RConn1 -- Diode4/LConn1 -- PV module 1/RConn2 -- Diode18/RConn1 -- PV module 15/RConn1 -- Diode3/RConn1 -- PV module 18/RConn1 -- Diode10/LConn1 -- PV module 7/RConn2 -- Diode7/LConn1 -- PV module 4/RConn2 -- Diode15/RConn1 -- PV module 12/RConn1 -- Diode29/LConn1 -- PV module 52/RConn2 -- Diode34/RConn1 -- PV module 31/RConn1 -- Diode64/RConn1 -- PV module 61/RConn1 -- Diode76/LConn1 -- PV module 55/RConn2 -- Diode61/RConn1 -- PV module 58/RConn1 -- Diode79/LConn1 -- PV module 76/RConn2
  Diode67/LConn1 -- PV module 73/RConn2 -- Diode65/RConn1 -- PV module 72/RConn1 -- PV module 40/RConn2 -- Diode43/LConn1 -- Diode46/LConn1 -- PV module 43/RConn2 -- Diode38/RConn1 -- PV module 45/RConn1 -- Diode40/LConn1 -- PV module 46/RConn2 -- PV module 19/RConn1 -- Diode22/RConn1 -- Diode25/RConn1 -- PV module 22/RConn1 -- Diode26/LConn1 -- PV module 23/RConn2 -- PV module 25/RConn1 -- Diode19/RConn1 -- PV module 26/RConn2 -- Diode20/LConn1 -- PV module 20/RConn2 -- Diode23/LConn1 -- Diode45/RConn1 -- PV module 42/RConn1 -- PV module 38/RConn1 -- Diode42/RConn1 -- Diode72/RConn1 -- PV module 69/RConn1 -- PV module 67/RConn2 -- Diode70/LConn1 -- Diode69/RConn1 -- PV module 65/RConn1 -- Diode73/LConn1 -- PV module 70/RConn2

== system power_PVArray_PartialShading9x9new/Double click here for more info ==

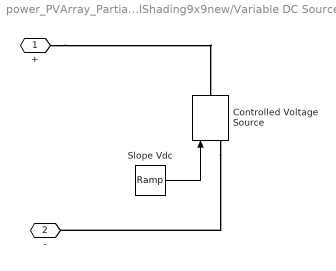
== system power_PVArray_PartialShading9x9new/Variable DC Source1 ==
  Controlled Voltage Source : powerlib/Electrical Sources/Controlled Voltage Source  Initialize=on  Source_Type=AC  Amplitude=0  Phase=0  Frequency=0  Measurements=None
      settings: SourceProductName=Simscape Electrical
  Slope Vdc : simulink/Sources/Ramp  slope=Slope_Vdc  start=0  InitialOutput=0
  + : PMIOPort  Side=Left
  - : PMIOPort  Port=2  Side=Left
  wires:
  Slope Vdc/1 -> Controlled Voltage Source/1
  connections:
  Controlled Voltage Source/LConn1 -- -/RConn1
  +/RConn1 -- Controlled Voltage Source/RConn1
